simulink model "GCU_clutch_model_tester"  (R2018a)
settings: Solver=FixedStepAuto  StartTime=0.0  StopTime=2  FixedStep=0.001  RelTol=1e-3
undefined symbols (not defined in the file): DiscIntNeverNeededParam, p
libraries: cstblocks x5, simulink x3
settings Model: Creator=Salvatore  LastModifiedBy=SIMONE

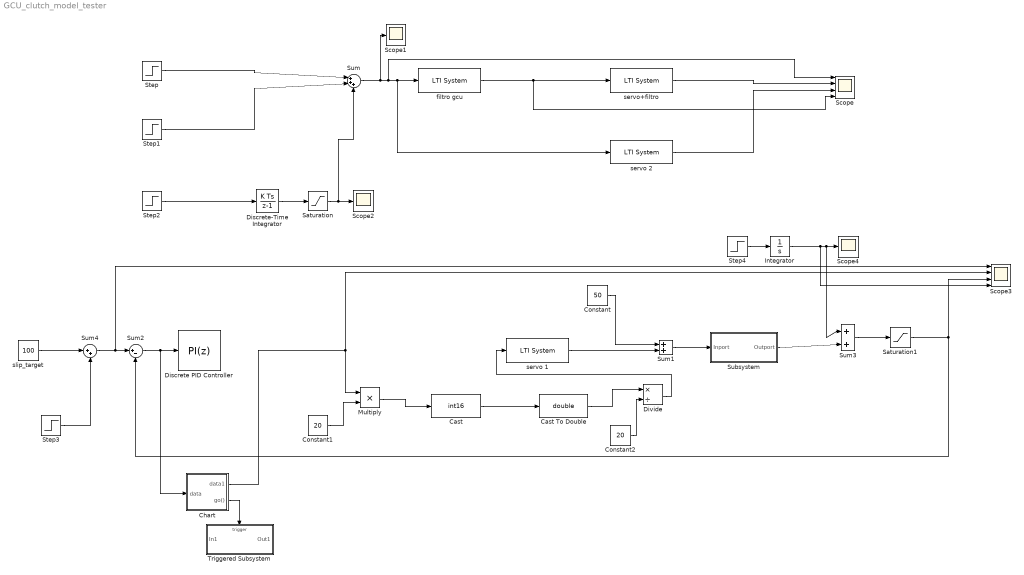
== system GCU_clutch_model_tester ==
  Cast : DataTypeConversion  OutDataTypeStr=int16
  Cast To Double : DataTypeConversion  OutDataTypeStr=double
  Chart : Stateflow chart  TreatAsAtomicUnit=on  SystemSampleTime=0.001
  Constant : Constant  Value=50  OutDataTypeStr=uint8
  Constant1 : Constant  Value=20  OutDataTypeStr=double
  Constant2 : Constant  Value=20  OutDataTypeStr=double
  Discrete PID Controller : simulink/Continuous/PID Controller  Controller=PI  TimeDomain=Discrete-time  SampleTime=0.01  IntegratorMethod=Forward Euler  FilterMethod=Forward Euler  Form=Parallel  UseFilter=on  ControllerParametersSource=internal  P=-0.52535095568031  I=-9.79580592329006  D=0.00664206143376672  N=13.2886258278716  InitialConditionSource=internal  InitialConditionForIntegrator=0  InitialConditionForFilter=0  ExternalReset=none  LimitOutput=on  UpperSaturationLimit=0  LowerSaturationLimit=-50  LinearizeAsGain=off  AntiWindupMode=back-calculation  Kb=1  TrackingMode=off  Kt=1  PParamMin=[]  PParamMax=[]  IParamMin=[]  IParamMax=[]  DParamMin=[]  DParamMax=[]  NParamMin=[]  NParamMax=[]  KbParamMin=[]  KbParamMax=[]  KtParamMin=[]  KtParamMax=[]  POutMin=[]  POutMax=[]  IOutMin=[]  IOutMax=[]  DOutMin=[]  DOutMax=[]  NOutMin=[]  NOutMax=[]  KbOutMin=[]  KbOutMax=[]  KtOutMin=[]  KtOutMax=[]  IntegratorOutMin=[]  IntegratorOutMax=[]  FilterOutMin=[]  FilterOutMax=[]  SumOutMin=[]  SumOutMax=[]  SumI1OutMin=[]  SumI1OutMax=[]  SumI2OutMin=[]  SumI2OutMax=[]  SumI3OutMin=[]  SumI3OutMax=[]  SumDOutMin=[]  SumDOutMax=[]  SaturationOutMin=[]  SaturationOutMax=[]  IntegratorContinuousStateAttributes=''  IntegratorStateMustResolveToSignalObject=off  IntegratorRTWStateStorageClass=Auto  FilterContinuousStateAttributes=''  FilterStateMustResolveToSignalObject=off  FilterRTWStateStorageClass=Auto  DifferentiatorICPrevScaledInput=0  DifferentiatorOutMin=[]  DifferentiatorOutMax=[]  FilterDiffOutCoefMin=[]  FilterDiffOutCoefMax=[]  SumDenOutMin=[]  SumDenOutMax=[]  SumNumOutMin=[]  SumNumOutMax=[]  ReciprocalOutMin=[]  ReciprocalOutMax=[]  DivideOutMin=[]  DivideOutMax=[]  TunerSelectOption=Transfer Function Based (PID Tuner App)
  Discrete-Time Integrator : DiscreteIntegrator  InitialCondition=50  SampleTime=0.025  ICPrevOutput=DiscIntNeverNeededParam  ICPrevScaledInput=DiscIntNeverNeededParam
  Divide : Product  Inputs=*/
  Integrator : Integrator
  Multiply : Product
  Saturation : Saturate  UpperLimit=100  LowerLimit=0  ZeroCross=off
  Saturation1 : Saturate  UpperLimit=100  LowerLimit=0  ZeroCross=off
  Scope : Scope  NumInputPorts=4
  Scope1 : Scope
  Scope2 : Scope
  Scope3 : Scope  NumInputPorts=4
  Scope4 : Scope
  Step : Step  Time=3  After=-50  SampleTime=0
  Step1 : Step  Time=0  After=50  SampleTime=0
  Step2 : Step  Time=3  After=-5/0.025  SampleTime=0
  Step3 : Step  Time=0.2  After=-93  SampleTime=0
  Step4 : Step  Time=0.6  After=-100  SampleTime=0
  Subsystem : Subsystem
  Sum : Sum  Inputs=|+++
  Sum1 : Sum
  Sum2 : Sum  Inputs=|+-
  Sum3 : Sum  Inputs=|++
  Sum4 : Sum  Inputs=|++
  Triggered Subsystem : Subsystem  TreatAsAtomicUnit=on
  filtro gcu : cstblocks/LTI System  sys=F_z  IC=[]
  servo 1 : cstblocks/LTI System  sys=g  IC=[]
  servo 2 : cstblocks/LTI System  sys=g  IC=[]
  servo+filtro : cstblocks/LTI System  sys=g  IC=[]
  slip_target : Constant  Value=100  OutDataTypeStr=uint8
  wires:
  filtro gcu/1 -> Scope/4, servo+filtro/1
  servo+filtro/1 -> Scope/2
  Sum/1 -> Scope1/1, Scope/1, servo 2/1, filtro gcu/1
  servo 2/1 -> Scope/3
  Discrete-Time Integrator/1 -> Saturation/1
  Saturation/1 -> Sum/3, Scope2/1
  Step2/1 -> Discrete-Time Integrator/1
  Step/1 -> Sum/1
  Step1/1 -> Sum/2
  Chart/1(data1) -> Multiply/1, Scope3/2
  Sum2/1 -> Chart/1(data), Discrete PID Controller/1
  servo 1/1 -> Sum1/2
  Constant/1 -> Sum1/1
  Sum1/1 -> Subsystem/1(Inport)
  Subsystem/1(Outport) -> Sum3/2
  Cast/1 -> Cast To Double/1
  Constant1/1 -> Multiply/2
  Multiply/1 -> Cast/1
  Constant2/1 -> Divide/2
  Cast To Double/1 -> Divide/1
  Divide/1 -> servo 1/1
  Step3/1 -> Sum4/2
  slip_target/1 -> Sum4/1
  Sum4/1 -> Scope3/1, Sum2/1
  Sum3/1 -> Saturation1/1
  Step4/1 -> Integrator/1
  Integrator/1 -> Scope3/4, Sum3/1, Scope4/1
  Saturation1/1 -> Sum2/2, Scope3/3
  Chart/2(go()) -> Triggered Subsystem/Trigger

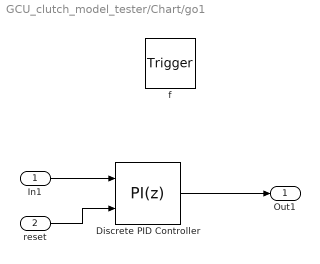
== system GCU_clutch_model_tester/Chart/go1 ==
  In1 : Inport  OutDataTypeStr=double  PortDimensions=1
  reset : Inport  Port=2  OutDataTypeStr=double  PortDimensions=1
  f : TriggerPort  TriggerType=function-call  VariantControl=(inherit)
      settings: CopyFcn=Stateflow.SLINSF.SimulinkMan.removeBlockPreDeleteFcn  PreDeleteFcn=Stateflow.SLINSF.SimulinkMan.unsafePredeleteFcn
  Discrete PID Controller : simulink/Continuous/PID Controller  Controller=PI  TimeDomain=Discrete-time  SampleTime=-1  IntegratorMethod=Forward Euler  FilterMethod=Forward Euler  Form=Parallel  UseFilter=on  ControllerParametersSource=internal  P=-0.52535095568031  I=-9.79580592329006  D=0.00664206143376672  N=13.2886258278716  InitialConditionSource=internal  InitialConditionForIntegrator=0  InitialConditionForFilter=0  ExternalReset=rising  LimitOutput=on  UpperSaturationLimit=0  LowerSaturationLimit=-50  LinearizeAsGain=off  AntiWindupMode=back-calculation  Kb=1  TrackingMode=off  Kt=1  PParamMin=[]  PParamMax=[]  IParamMin=[]  IParamMax=[]  DParamMin=[]  DParamMax=[]  NParamMin=[]  NParamMax=[]  KbParamMin=[]  KbParamMax=[]  KtParamMin=[]  KtParamMax=[]  POutMin=[]  POutMax=[]  IOutMin=[]  IOutMax=[]  DOutMin=[]  DOutMax=[]  NOutMin=[]  NOutMax=[]  KbOutMin=[]  KbOutMax=[]  KtOutMin=[]  KtOutMax=[]  IntegratorOutMin=[]  IntegratorOutMax=[]  FilterOutMin=[]  FilterOutMax=[]  SumOutMin=[]  SumOutMax=[]  SumI1OutMin=[]  SumI1OutMax=[]  SumI2OutMin=[]  SumI2OutMax=[]  SumI3OutMin=[]  SumI3OutMax=[]  SumDOutMin=[]  SumDOutMax=[]  SaturationOutMin=[]  SaturationOutMax=[]  IntegratorContinuousStateAttributes=''  IntegratorStateMustResolveToSignalObject=off  IntegratorRTWStateStorageClass=Auto  FilterContinuousStateAttributes=''  FilterStateMustResolveToSignalObject=off  FilterRTWStateStorageClass=Auto  DifferentiatorICPrevScaledInput=0  DifferentiatorOutMin=[]  DifferentiatorOutMax=[]  FilterDiffOutCoefMin=[]  FilterDiffOutCoefMax=[]  SumDenOutMin=[]  SumDenOutMax=[]  SumNumOutMin=[]  SumNumOutMax=[]  ReciprocalOutMin=[]  ReciprocalOutMax=[]  DivideOutMin=[]  DivideOutMax=[]  TunerSelectOption=Frequency Response Based
  Out1 : Outport  OutDataTypeStr=double  PortDimensions=1
  wires:
  Discrete PID Controller/1 -> Out1/1
  In1/1 -> Discrete PID Controller/1
  reset/1 -> Discrete PID Controller/2

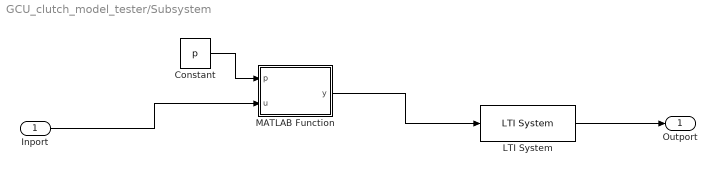
== system GCU_clutch_model_tester/Subsystem ==
  Inport : Inport
  Constant : Constant  Value=p  OutDataTypeStr=double
  LTI System : cstblocks/LTI System  sys=d  IC=[]
  MATLAB Function : MATLAB Function  TreatAsAtomicUnit=on
  Outport : Outport
  wires:
  Inport/1 -> MATLAB Function/2(u)
  LTI System/1 -> Outport/1
  Constant/1 -> MATLAB Function/1(p)
  MATLAB Function/1(y) -> LTI System/1

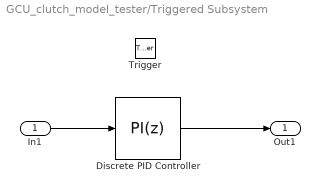
== system GCU_clutch_model_tester/Triggered Subsystem ==
  In1 : Inport
  Trigger : TriggerPort  TriggerType=function-call  VariantControl=Variant
  Discrete PID Controller : simulink/Continuous/PID Controller  Controller=PI  TimeDomain=Discrete-time  SampleTime=-1  IntegratorMethod=Forward Euler  FilterMethod=Forward Euler  Form=Parallel  UseFilter=on  ControllerParametersSource=internal  P=-0.52535095568031  I=-9.79580592329006  D=0.00664206143376672  N=13.2886258278716  InitialConditionSource=internal  InitialConditionForIntegrator=0  InitialConditionForFilter=0  ExternalReset=none  LimitOutput=on  UpperSaturationLimit=0  LowerSaturationLimit=-50  LinearizeAsGain=off  AntiWindupMode=back-calculation  Kb=1  TrackingMode=off  Kt=1  PParamMin=[]  PParamMax=[]  IParamMin=[]  IParamMax=[]  DParamMin=[]  DParamMax=[]  NParamMin=[]  NParamMax=[]  KbParamMin=[]  KbParamMax=[]  KtParamMin=[]  KtParamMax=[]  POutMin=[]  POutMax=[]  IOutMin=[]  IOutMax=[]  DOutMin=[]  DOutMax=[]  NOutMin=[]  NOutMax=[]  KbOutMin=[]  KbOutMax=[]  KtOutMin=[]  KtOutMax=[]  IntegratorOutMin=[]  IntegratorOutMax=[]  FilterOutMin=[]  FilterOutMax=[]  SumOutMin=[]  SumOutMax=[]  SumI1OutMin=[]  SumI1OutMax=[]  SumI2OutMin=[]  SumI2OutMax=[]  SumI3OutMin=[]  SumI3OutMax=[]  SumDOutMin=[]  SumDOutMax=[]  SaturationOutMin=[]  SaturationOutMax=[]  IntegratorContinuousStateAttributes=''  IntegratorStateMustResolveToSignalObject=off  IntegratorRTWStateStorageClass=Auto  FilterContinuousStateAttributes=''  FilterStateMustResolveToSignalObject=off  FilterRTWStateStorageClass=Auto  DifferentiatorICPrevScaledInput=0  DifferentiatorOutMin=[]  DifferentiatorOutMax=[]  FilterDiffOutCoefMin=[]  FilterDiffOutCoefMax=[]  SumDenOutMin=[]  SumDenOutMax=[]  SumNumOutMin=[]  SumNumOutMax=[]  ReciprocalOutMin=[]  ReciprocalOutMax=[]  DivideOutMin=[]  DivideOutMax=[]  TunerSelectOption=Transfer Function Based (PID Tuner App)
  Out1 : Outport
  wires:
  In1/1 -> Discrete PID Controller/1
  Discrete PID Controller/1 -> Out1/1

== matlab function GCU_clutch_model_tester/Subsystem/MATLAB Function ==
  data: p input; u input; y output
function y = calcoloSlip(p,u)

y = polyval(p,u);

== stateflow chart GCU_clutch_model_tester/Chart ==
  state c
    data1=go1(data,1);
  state b
    entry:counter = 1;
    during: counter = counter + 1;
  state a
    entry:send(go);
    data1=go1(data,0);
  state Out1 = go1(In1,reset) [function]
  (default) -> c
  c -> a
  b -> a : [counter>=9]
  a -> b
  data: In1 function_input double size=1; Out1 function_output double size=1; reset function_input double size=1; counter local; data input; data1 output =0
  events: go output FUNCTION_CALL_EVENT
